simulink model "Vehicle_Model_999_Modular_roll_gradient"  (R2025b)
settings: Solver=ode23tb  StartTime=0.0  StopTime=72  MaxStep=0.001  RelTol=1e-3
values from neighbouring files (symbols this model uses):
  aero_par = struct()    [Load_aero_parameters.m]
  Ki_array = zeros(size(Vx_array))    [Torque_vectoring_workspace_lookuptable_v2.m]
  Kp_array = zeros(size(Vx_array))    [Torque_vectoring_workspace_lookuptable_v2.m]
  ku = (lr*m*9.81/(cf*(lf+lr))) - (lf*m*9.81/(cr*(lf+lr)))    (= -0.00172747958109)    [Torque_vectoring_workspace_lookuptable_v2.m]
  m = Par.m    [Lapsim_Endurance_inverse_v3.m]    (also in New_LapSim_final_ts_v1.m = Par.Mass; Rajdeep_sus_scriptv2.m = 270; Torque_vectoring_workspace_lookuptable_v2.m = 270)
  Par = struct()    [Load_vehicle_parameters.m]
  path_Theta = theta-theta_0    [New_LapSim_final_ts_v1.m]
  sus_par = struct()    [Load_sus_parameters.m]
  TireData = Tir    [prep_tire_data.m]
  Vx_array = 1:1:21    [Torque_vectoring_workspace_lookuptable_v2.m]
undefined symbols (not defined in the file or in its folder): additional_steering, Battery, Brake_Val, ctrl_Brake, ctrl_s, ctrl_Steer, ctrl_Throttle, ctrl_Velocity, HP, init_r, init_vx, init_vy, Motor, path_X, path_Y, skidpad_time, skidpad_vel, steer_input, Steer_Val, TC_target_slip, Throttle_Val, V_ref
libraries: simulink x16, autolibshared x3, simulink_extras x2, BatteryEstimators x1
(part 2 of 4)

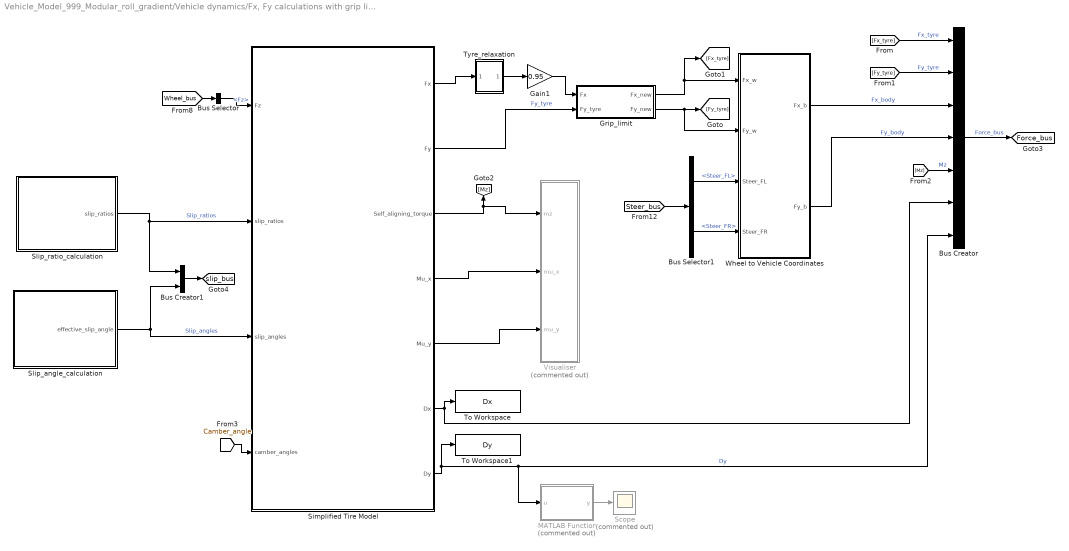
== system Vehicle_Model_999_Modular_roll_gradient/Vehicle dynamics/Fx, Fy calculations with grip limit ==
  Bus Creator : BusCreator  Inputs=7
  Bus Creator1 : BusCreator  Inputs=2
  Bus Selector : BusSelector  OutputSignals=Fz
  Bus Selector1 : BusSelector  OutputSignals=Steer_FL,Steer_FR
  Gain1 : Gain  Gain=0.95
  Grip_limit : Subsystem
  MATLAB Function : MATLAB Function  Commented=on  TreatAsAtomicUnit=on
  Scope : Scope  Commented=on
      settings: ActiveDisplayYMinimum=-1  ActiveDisplayYMaximum=1  DataLoggingVariableName=ScopeData16
  Simplified Tire Model : MATLAB Function  TreatAsAtomicUnit=on
  Slip_angle_calculation : Subsystem
  Slip_ratio_calculation : Subsystem
  To Workspace : ToWorkspace  VariableName=Dx  SaveFormat=Timeseries  SampleTime=-1
  To Workspace1 : ToWorkspace  VariableName=Dy  SaveFormat=Timeseries  SampleTime=-1
  Tyre_relaxation : Subsystem
  Visualiser : Subsystem  Commented=on
  Wheel to Vehicle Coordinates : MATLAB Function  TreatAsAtomicUnit=on
  tag scope: Force_bus=global, slip_bus=global
  wires:
  Simplified Tire Model/1(Fx) -> Tyre_relaxation/1(Fx_ss)
  Simplified Tire Model/6(Dx) -> To Workspace/1, Bus Creator/6
  [Wheel_bus] -> Bus Selector/1
  Bus Selector/1 -> Simplified Tire Model/1(Fz)  "<Fz>"
  Bus Creator1/1 -> [slip_bus]
  Bus Creator/1 -> [Force_bus]  "Force_bus"
  [Mz] -> Bus Creator/5  "Mz"
  [Fx_tyre] -> Bus Creator/1  "Fx_tyre"
  [Fy_tyre] -> Bus Creator/2  "Fy_tyre"
  Slip_ratio_calculation/1(slip_ratios) -> Simplified Tire Model/2(slip_ratios), Bus Creator1/1  "Slip_ratios"
  Slip_angle_calculation/1(effective_slip_angle) -> Simplified Tire Model/3(slip_angles), Bus Creator1/2  "Slip_angles"
  Bus Selector1/2 -> Wheel to Vehicle Coordinates/4(Steer_FR)  "<Steer_FR>"
  [Steer_bus] -> Bus Selector1/1
  Simplified Tire Model/4(Mu_x) -> Visualiser/2(mu_x)
  Wheel to Vehicle Coordinates/1(Fx_b) -> Bus Creator/3  "Fx_body"
  Simplified Tire Model/5(Mu_y) -> Visualiser/3(mu_y)
  Bus Selector1/1 -> Wheel to Vehicle Coordinates/3(Steer_FL)  "<Steer_FL>"
  Simplified Tire Model/7(Dy) -> MATLAB Function/1(u), Bus Creator/7, To Workspace1/1  "Dy"
  Tyre_relaxation/1(Fx_w) -> Gain1/1
  Simplified Tire Model/3(Self_aligning_torque) -> Visualiser/1(mz), [Mz]
  Wheel to Vehicle Coordinates/2(Fy_b) -> Bus Creator/4  "Fy_body"
  [Camber_angle] -> Simplified Tire Model/4(camber_angles)
  MATLAB Function/1(y) -> Scope/1
  Grip_limit/2(Fy_new) -> Wheel to Vehicle Coordinates/2(Fy_w), [Fy_tyre]
  Grip_limit/1(Fx_new) -> [Fx_tyre], Wheel to Vehicle Coordinates/1(Fx_w)
  Gain1/1 -> Grip_limit/1(Fx)
  Simplified Tire Model/2(Fy) -> Grip_limit/2(Fy_tyre)  "Fy_tyre"

== system Vehicle_Model_999_Modular_roll_gradient/Vehicle dynamics/Rolling and Drag forces ==
  Aero Drag : MATLAB Function  TreatAsAtomicUnit=on
  Bus Creator : BusCreator  Inputs=3
  Bus Selector : BusSelector  OutputSignals=Fz
  Bus Selector1 : BusSelector  OutputSignals=Steer_FL,Steer_FR
  Bus Selector2 : BusSelector  OutputSignals=Longitudinal_vel,Lateral_vel
  MATLAB Function : MATLAB Function  TreatAsAtomicUnit=on
  Rolling Forces : MATLAB Function  TreatAsAtomicUnit=on
  Terminator : Terminator
  To Workspace : ToWorkspace  Commented=on  VariableName=Dragforce  SaveFormat=Timeseries  SampleTime=-1
  tag scope: Resistive_force_bus=global
  wires:
  Bus Selector1/1 -> Rolling Forces/2(Steer_FL)  "<Steer_FL>"
  Bus Selector2/1 -> Aero Drag/1(vx)  "<Longitudinal_vel>"
  Bus Selector/1 -> Rolling Forces/1(Fz)  "<Fz>"
  Aero Drag/1(B_F_aero) -> MATLAB Function/1(u), Bus Creator/3  "Aero_drag_force"
  Rolling Forces/1(Fx_rr_b) -> Bus Creator/1  "Longitudinal_rolling_resistance"
  Bus Selector1/2 -> Rolling Forces/3(Steer_FR)  "<Steer_FR>"
  Bus Selector2/2 -> Aero Drag/2(vy)  "<Lateral_vel>"
  Rolling Forces/2(Fy_rr_b) -> Bus Creator/2  "Lateral_rolling_resistance"
  Bus Creator/1 -> [Resistive_force_bus]
  MATLAB Function/1(y) -> To Workspace/1, Terminator/1  "Drag_force"
  [Wheel_bus] -> Bus Selector/1
  [Steer_bus] -> Bus Selector1/1
  [chassisbus] -> Bus Selector2/1

== system Vehicle_Model_999_Modular_roll_gradient/Vehicle dynamics/Steering ==
  Bus Selector12 : BusSelector  OutputSignals=Steer_input
  Constant1 : Constant  Value=sus_par.Acc_pct
  Steering Kinematics : Subsystem
  tag scope: Steer_bus=global
  wires:
  Bus Selector12/1 -> Steering Kinematics/1(Steer_Input)  "<Steer_input>"
  Constant1/1 -> Steering Kinematics/2(Ackermann_Pct)
  [Input_bus] -> Bus Selector12/1
  Steering Kinematics/1(Steering Angles) -> [Steer_bus]

== system Vehicle_Model_999_Modular_roll_gradient/Vehicle dynamics/Steering_new ==
  Bus Creator1 : BusCreator  Inputs=2
  Bus Selector12 : BusSelector  OutputSignals=Steer_input
  Display : Display  Commented=on
  Display1 : Display  Commented=on
  Steering Kinematics : MATLAB Function  TreatAsAtomicUnit=on
  To Workspace : ToWorkspace  VariableName=steer_L  SaveFormat=Timeseries  SampleTime=-1
  To Workspace1 : ToWorkspace  VariableName=steer_R  SaveFormat=Timeseries  SampleTime=-1
  tag scope: Steer_bus=global
  wires:
  Bus Creator1/1 -> [Steer_bus]
  [Input_bus] -> Bus Selector12/1
  Bus Selector12/1 -> Steering Kinematics/1(steering_wheel_angle)  "<Steer_input>"
  Steering Kinematics/2(Steer_R) -> Display/1, To Workspace1/1, Bus Creator1/2  "Steer_FR"
  Steering Kinematics/1(Steer_L) -> Display1/1, To Workspace/1, Bus Creator1/1  "Steer_FL"

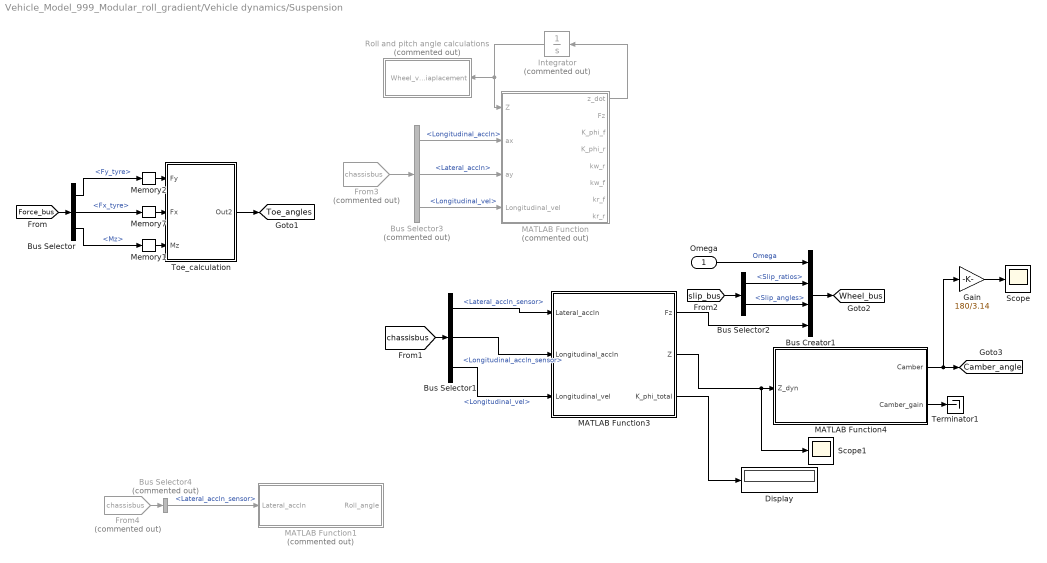
== system Vehicle_Model_999_Modular_roll_gradient/Vehicle dynamics/Suspension ==
  Omega : Inport
  Bus Creator1 : BusCreator  Inputs=4
  Bus Selector : BusSelector  OutputSignals=Fy_tyre,Fx_tyre,Mz
  Bus Selector1 : BusSelector  OutputSignals=Lateral_accln_sensor,Longitudinal_accln_sensor,Longitudinal_vel
  Bus Selector2 : BusSelector  OutputSignals=Slip_ratios,Slip_angles
  Bus Selector3 : BusSelector  Commented=on  OutputSignals=Longitudinal_accln,Lateral_accln,Longitudinal_vel
  Bus Selector4 : BusSelector  Commented=on  OutputSignals=Lateral_accln_sensor
  Display : Display
  From3 : From  Commented=on  GotoTag=chassisbus  TagVisibility=global
  From4 : From  Commented=on  GotoTag=chassisbus  TagVisibility=global
  Gain : Gain  Gain=180/3.14
  Integrator : Integrator  Commented=on
  MATLAB Function : MATLAB Function  Commented=on  TreatAsAtomicUnit=on
  MATLAB Function1 : MATLAB Function  Commented=on  TreatAsAtomicUnit=on
  MATLAB Function3 : MATLAB Function  TreatAsAtomicUnit=on
  MATLAB Function4 : MATLAB Function  TreatAsAtomicUnit=on
  Memory1 : Memory
  Memory2 : Memory
  Memory7 : Memory
  Roll and pitch angle calculations : Subsystem  Commented=on
  Scope : Scope
      settings: ActiveDisplayYMinimum=-0.32429469761940044  ActiveDisplayYMaximum=0.29371949735728869  DataLoggingVariableName=ScopeData3
  Scope1 : Scope
      settings: ActiveDisplayYMinimum=-0.021192676708042583  ActiveDisplayYMaximum=0.035474266047541975  DataLoggingVariableName=ScopeData4
  Terminator1 : Terminator
  Toe_calculation : Subsystem
  tag scope: Camber_angle=global, Toe_angles=global, Wheel_bus=global
  wires:
  Toe_calculation/1(Out2) -> [Toe_angles]
  Memory7/1 -> Toe_calculation/2(Fx)
  Memory1/1 -> Toe_calculation/3(Mz)
  Memory2/1 -> Toe_calculation/1(Fy)
  Bus Selector/1 -> Memory2/1  "<Fy_tyre>"
  [Force_bus] -> Bus Selector/1
  Bus Selector/2 -> Memory7/1  "<Fx_tyre>"
  Bus Selector/3 -> Memory1/1  "<Mz>"
  Omega/1 -> Bus Creator1/1  "Omega"
  Bus Selector2/2 -> Bus Creator1/3  "<Slip_angles>"
  From3/1 -> Bus Selector3/1
  Bus Selector3/1 -> MATLAB Function/2(ax)  "<Longitudinal_accln>"
  Bus Selector2/1 -> Bus Creator1/2  "<Slip_ratios>"
  Bus Selector3/2 -> MATLAB Function/3(ay)  "<Lateral_accln>"
  Bus Creator1/1 -> [Wheel_bus]
  [slip_bus] -> Bus Selector2/1
  Integrator/1 -> Roll and pitch angle calculations/1(Wheel_vertical_diaplacement), MATLAB Function/1(Z)
  Bus Selector3/3 -> MATLAB Function/4(Longitudinal_vel)  "<Longitudinal_vel>"
  MATLAB Function3/1(Fz) -> Bus Creator1/4
  [chassisbus] -> Bus Selector1/1
  Bus Selector1/3 -> MATLAB Function3/3(Longitudinal_vel)  "<Longitudinal_vel>"
  MATLAB Function4/1(Camber) -> Gain/1, [Camber_angle]
  MATLAB Function4/2(Camber_gain) -> Terminator1/1
  MATLAB Function3/2(Z) -> Scope1/1, MATLAB Function4/1(Z_dyn)
  MATLAB Function/1(z_dot) -> Integrator/1
  Bus Selector1/1 -> MATLAB Function3/1(Lateral_accln)  "<Lateral_accln_sensor>"
  Bus Selector1/2 -> MATLAB Function3/2(Longitudinal_accln)  "<Longitudinal_accln_sensor>"
  From4/1 -> Bus Selector4/1
  Bus Selector4/1 -> MATLAB Function1/1(Lateral_accln)  "<Lateral_accln_sensor>"
  Gain/1 -> Scope/1
  MATLAB Function3/3(K_phi_total) -> Display/1

== system Vehicle_Model_999_Modular_roll_gradient/Vehicle dynamics/Wheel_dynamics ==
  Bus Selector13 : BusSelector  OutputSignals=Fz
  Bus Selector14 : BusSelector  OutputSignals=Slip_angles
  Bus Selector30 : BusSelector  OutputSignals=Omega
  Rolling Resistance : MATLAB Function  TreatAsAtomicUnit=on
  Wheel Dynamics : Subsystem
  Omega1 : Outport
  wires:
  [Wheel_bus] -> Bus Selector14/1, Bus Selector30/1, Bus Selector13/1
  Bus Selector30/1 -> Rolling Resistance/2(Omega)  "<Omega>"
  Rolling Resistance/1(wFx_rr) -> Wheel Dynamics/1(Fx_rr)
  Bus Selector13/1 -> Rolling Resistance/1(Fz)  "<Fz>"
  Bus Selector14/1 -> Rolling Resistance/3(slip_angles)  "<Slip_angles>"
  Wheel Dynamics/1(Omega) -> Omega1/1

== system Vehicle_Model_999_Modular_roll_gradient/Visualization/Visualize Fx ==
  Fx_tire : Inport
  Demux : Demux
  To Workspace : ToWorkspace  VariableName=Longitudinal_force_fl  SaveFormat=Timeseries  SampleTime=-1
  To Workspace1 : ToWorkspace  VariableName=Longitudinal_force_fr  SaveFormat=Timeseries  SampleTime=-1
  To Workspace2 : ToWorkspace  VariableName=Longitudinal_force_rl  SaveFormat=Timeseries  SampleTime=-1
  To Workspace3 : ToWorkspace  VariableName=Longitudinal_force_rr  SaveFormat=Timeseries  SampleTime=-1
  Visualize_longitudinal_force_tire : Scope  Commented=on  NumInputPorts=4
      settings: ActiveDisplayYMinimum=-744.61831418304712  ActiveDisplayYMaximum=150.84371621033421  DataLoggingVariableName=ScopeData2
  wires:
  Fx_tire/1 -> Demux/1
  Demux/1 -> To Workspace/1, Visualize_longitudinal_force_tire/1  "Longitudinal_force_fl"
  Demux/2 -> To Workspace1/1, Visualize_longitudinal_force_tire/2  "Longitudinal_force_fr"
  Demux/3 -> To Workspace2/1, Visualize_longitudinal_force_tire/3  "Longitudinal_force_rl"
  Demux/4 -> To Workspace3/1, Visualize_longitudinal_force_tire/4  "Longitudinal_force_rr"

== system Vehicle_Model_999_Modular_roll_gradient/Visualization/Visualize Fy ==
  Fy_tire : Inport
  Demux : Demux
  To Workspace1 : ToWorkspace  VariableName=Lateral_force_fl  SaveFormat=Timeseries  SampleTime=-1
  To Workspace2 : ToWorkspace  VariableName=Lateral_force_fr  SaveFormat=Timeseries  SampleTime=-1
  To Workspace3 : ToWorkspace  VariableName=Lateral_force_rl  SaveFormat=Timeseries  SampleTime=-1
  To Workspace4 : ToWorkspace  VariableName=Lateral_force_rr  SaveFormat=Timeseries  SampleTime=-1
  Visualize_lateral_force_tire : Scope  Commented=on  NumInputPorts=4
      settings: ActiveDisplayYMinimum=-149.71186810034453  ActiveDisplayYMaximum=870.76288445594662  DataLoggingVariableName=ScopeData2
  wires:
  Demux/4 -> To Workspace4/1, Visualize_lateral_force_tire/4  "Lateral_force_rr"
  Demux/3 -> To Workspace3/1, Visualize_lateral_force_tire/3  "Lateral_force_rl"
  Demux/2 -> To Workspace2/1, Visualize_lateral_force_tire/2  "Lateral_force_fr"
  Demux/1 -> To Workspace1/1, Visualize_lateral_force_tire/1  "Lateral_force_fl"
  Fy_tire/1 -> Demux/1

== system Vehicle_Model_999_Modular_roll_gradient/Visualization/Visualize Fz ==
  Fz : Inport
  Demux : Demux
  To Workspace : ToWorkspace  VariableName=Fz  SaveFormat=Timeseries  SampleTime=-1
  Visualize_Fz : Scope  Commented=on  NumInputPorts=4
      settings: ActiveDisplayYMinimum=-105.77095780933836  ActiveDisplayYMaximum=951.93862028404544  DataLoggingVariableName=ScopeData2
  wires:
  Fz/1 -> Demux/1
  Demux/1 -> To Workspace/1, Visualize_Fz/1  "Fz_fl"
  Demux/2 -> Visualize_Fz/2  "Fz_fr"
  Demux/3 -> Visualize_Fz/3  "Fz_rl"
  Demux/4 -> Visualize_Fz/4  "Fz_rr"

== system Vehicle_Model_999_Modular_roll_gradient/E-powertrain/Battery Pack/Subsystem ==
  In1 : Inport
  Constant : Constant  Value=0.001
  Switch : Switch  Criteria=u2 > Threshold  SaturateOnIntegerOverflow=off  InputSameDT=off
  Out1 : Outport
  wires:
  In1/1 -> Switch/1, Switch/2
  Constant/1 -> Switch/3
  Switch/1 -> Out1/1

== system Vehicle_Model_999_Modular_roll_gradient/E-powertrain/Torque Distribution/Torque Vectoring ==
  steering angle : Inport
  vx : Inport  Port=2
  real yaw rate : Inport  Port=3
  Wheel Torques : Inport  Port=4
  1-D Lookup Table1 : Lookup_n-D  NumberOfTableDimensions=1  BreakpointsForDimension1=Vx_array  Table=Kp_array  InternalRulePriority=Speed  RndMeth=Simplest
  1-D Lookup Table2 : Lookup_n-D  NumberOfTableDimensions=1  BreakpointsForDimension1=Vx_array  Table=Ki_array  InternalRulePriority=Speed  RndMeth=Simplest
  MATLAB Function : MATLAB Function  TreatAsAtomicUnit=on
  MATLAB Function1 : MATLAB Function  TreatAsAtomicUnit=on
  PID controller in time domain : MATLAB Function  TreatAsAtomicUnit=on  SystemSampleTime=0.001
  Target yaw rate : Subsystem
  To Workspace : ToWorkspace  VariableName=Target_yaw_rate  SaveFormat=Timeseries  SampleTime=-1
  Vectored Torque Commands : Outport
  wires:
  steering angle/1 -> Target yaw rate/1(steering angle)
  Wheel Torques/1 -> MATLAB Function/1(wheel_torques)
  MATLAB Function/1(vectored_torques) -> Vectored Torque Commands/1
  vx/1 -> 1-D Lookup Table2/1, 1-D Lookup Table1/1, Target yaw rate/2(vx)
  PID controller in time domain/1(yaw_moment) -> MATLAB Function/2(yaw_moment)
  real yaw rate/1 -> MATLAB Function1/1(u)
  MATLAB Function1/1(y) -> PID controller in time domain/2(y)
  1-D Lookup Table1/1 -> PID controller in time domain/3(Kp)
  1-D Lookup Table2/1 -> PID controller in time domain/4(Ki)
  Target yaw rate/1(target yaw rate) -> To Workspace/1, PID controller in time domain/1(ref)

== system Vehicle_Model_999_Modular_roll_gradient/E-powertrain/Torque Distribution/Traction Control ==
  Wheel Torque : Inport
  Slip Ratios : Inport  Port=2
  vx : Inport  Port=3
  Constant3 : Constant  Value=TC_target_slip
  KD1 : Lookup_n-D  NumberOfTableDimensions=1  BreakpointsForDimension1=[0, 55e-10, 0.0045, 2, 8.5,9]  Table=[0, 0, 0.0014, 0.0109,0,0]  InternalRulePriority=Speed  RndMeth=Simplest
  KI1 : Lookup_n-D  NumberOfTableDimensions=1  BreakpointsForDimension1=[0; 55e-10;0.0045; 2; 8.5]  Table=[0.1; 0.1;700; 500; 450 ]  InternalRulePriority=Speed  RndMeth=Simplest
  KP1 : Lookup_n-D  NumberOfTableDimensions=1  BreakpointsForDimension1=[0; 55e-10; 0.0045; 2; 8.5]  Table=[ 0.5; 0.5; 2.5; 10; 10]  InternalRulePriority=Speed  RndMeth=Simplest
  MATLAB Function1 : MATLAB Function  TreatAsAtomicUnit=on  SystemSampleTime=0.001
  MATLAB Function2 : MATLAB Function  TreatAsAtomicUnit=on
  Traction Controlled Torque : Outport
  wires:
  KD1/1 -> MATLAB Function1/5(Kd)
  KI1/1 -> MATLAB Function1/4(Ki)
  KP1/1 -> MATLAB Function1/3(Kp)
  vx/1 -> KD1/1, KI1/1, KP1/1
  Slip Ratios/1 -> MATLAB Function1/2(lambda_actual)
  Constant3/1 -> MATLAB Function1/1(lambda_ref)
  Wheel Torque/1 -> MATLAB Function2/2(torque_wheel)
  MATLAB Function1/1(throttle_cmd) -> MATLAB Function2/1(torque_pid)
  MATLAB Function2/1(TC_output) -> Traction Controlled Torque/1

== system Vehicle_Model_999_Modular_roll_gradient/E-powertrain/Torque Distribution/is TCS on? ==
  traction_controlled_torque : Inport
  In1 : Inport  Port=2
  TV_T_wheel : Inport  Port=3
  AND : Logic  IconShape=distinctive  AllPortsSameDT=off  OutDataTypeStr=boolean
  Bus Selector6 : BusSelector  OutputSignals=Steer_input
  MATLAB Function1 : MATLAB Function  TreatAsAtomicUnit=on
  Switch : Switch  Criteria=u2 > Threshold  SaturateOnIntegerOverflow=off  InputSameDT=off
  torque_output : Outport
  wires:
  Switch/1 -> torque_output/1
  TV_T_wheel/1 -> Switch/3
  traction_controlled_torque/1 -> Switch/1
  In1/1 -> AND/2
  AND/1 -> Switch/2
  Bus Selector6/1 -> MATLAB Function1/1(Steer_input)  "<Steer_input>"
  [Input_bus] -> Bus Selector6/1
  MATLAB Function1/1(TC_on) -> AND/1

== system Vehicle_Model_999_Modular_roll_gradient/E-powertrain/Torque Distribution/is TV on? ==
  vectored_torque : Inport
  In1 : Inport  Port=2
  wheel_torque : Inport  Port=3
  Switch : Switch  Criteria=u2 > Threshold  SaturateOnIntegerOverflow=off  InputSameDT=off
  torque_output : Outport
  wires:
  wheel_torque/1 -> Switch/3
  vectored_torque/1 -> Switch/1
  Switch/1 -> torque_output/1
  In1/1 -> Switch/2

== system Vehicle_Model_999_Modular_roll_gradient/Inputs/Brake_input_selector/Brake Variant Subsystem ==
  brake_sim : Inport
  vel : Inport  Port=2
  GGV : Subsystem  VariantControl=Mode_ggv
  Sideslip_vs_curvature_cst_accln : Subsystem  VariantControl=Mode_sideslip_vs_curvature_cst_accln
  Simulink : Subsystem  VariantControl=Mode_simulink
  curvature vs steer_angle : Subsystem  VariantControl=Mode_curvature_vs_steer
  sideslip_vs_curvature : Subsystem  VariantControl=Mode_sideslip_vs_curvature
  steerdiff_vs_ay : Subsystem  VariantControl=Mode_steerdiff_vs_ay
  timeseries : Subsystem  VariantControl=Mode_timeseries
  brake_input : Outport
  accln : Outport  Port=2

== system Vehicle_Model_999_Modular_roll_gradient/Inputs/Subsystem/Subsystem ==
  In1 : Inport
  Abs : Abs  SaturateOnIntegerOverflow=off
  Constant : Constant  Value=0.0001
  Switch : Switch  Criteria=u2 > Threshold  SaturateOnIntegerOverflow=off  InputSameDT=off
  Out1 : Outport
  wires:
  In1/1 -> Abs/1, Switch/1
  Constant/1 -> Switch/3
  Abs/1 -> Switch/2
  Switch/1 -> Out1/1

== system Vehicle_Model_999_Modular_roll_gradient/Inputs/Subsystem/Subsystem1 ==
  In1 : Inport
  Abs : Abs  SaturateOnIntegerOverflow=off
  Constant : Constant  Value=0.0001
  Switch : Switch  Criteria=u2 > Threshold  SaturateOnIntegerOverflow=off  InputSameDT=off
  Out1 : Outport
  wires:
  In1/1 -> Abs/1, Switch/1
  Constant/1 -> Switch/3
  Abs/1 -> Switch/2
  Switch/1 -> Out1/1

== system Vehicle_Model_999_Modular_roll_gradient/Inputs/Subsystem/Triggered Subsystem ==
  In1 : Inport
  Trigger : TriggerPort  VariantControl=(inherit)
  Out1 : Outport
  wires:
  In1/1 -> Out1/1

== system Vehicle_Model_999_Modular_roll_gradient/Inputs/Subsystem/Triggered Subsystem1 ==
  In1 : Inport
  Trigger : TriggerPort  VariantControl=(inherit)
  Out1 : Outport
  wires:
  In1/1 -> Out1/1

== system Vehicle_Model_999_Modular_roll_gradient/Inputs/Subsystem/Triggered Subsystem2 ==
  In1 : Inport
  Trigger : TriggerPort  VariantControl=(inherit)
  Out1 : Outport
  wires:
  In1/1 -> Out1/1

== system Vehicle_Model_999_Modular_roll_gradient/Inputs/Subsystem/Triggered Subsystem3 ==
  In1 : Inport
  In3 : Inport  Port=2
  Trigger : TriggerPort  VariantControl=(inherit)
  Out1 : Outport
  Out3 : Outport  Port=2
  wires:
  In1/1 -> Out1/1
  In3/1 -> Out3/1

== system Vehicle_Model_999_Modular_roll_gradient/Inputs/Subsystem/Triggered Subsystem4 ==
  In1 : Inport
  Trigger : TriggerPort  VariantControl=(inherit)
  Out1 : Outport
  wires:
  In1/1 -> Out1/1

== system Vehicle_Model_999_Modular_roll_gradient/Inputs/Subsystem/Triggered Subsystem5 ==
  In1 : Inport
  Trigger : TriggerPort  VariantControl=(inherit)
  Out1 : Outport
  wires:
  In1/1 -> Out1/1

== system Vehicle_Model_999_Modular_roll_gradient/Inputs/Subsystem/Triggered Subsystem6 ==
  In1 : Inport
  Trigger : TriggerPort  VariantControl=(inherit)
  Out1 : Outport
  wires:
  In1/1 -> Out1/1

== system Vehicle_Model_999_Modular_roll_gradient/Inputs/Subsystem1/Triggered Subsystem ==
  In1 : Inport
  Trigger : TriggerPort  VariantControl=(inherit)
  Out1 : Outport
  wires:
  In1/1 -> Out1/1

== system Vehicle_Model_999_Modular_roll_gradient/Inputs/Subsystem1/Triggered Subsystem1 ==
  In1 : Inport
  Trigger : TriggerPort  VariantControl=(inherit)
  Out1 : Outport
  wires:
  In1/1 -> Out1/1

== system Vehicle_Model_999_Modular_roll_gradient/Inputs/Subsystem1/Triggered Subsystem2 ==
  In1 : Inport
  Trigger : TriggerPort  VariantControl=(inherit)
  Out1 : Outport
  wires:
  In1/1 -> Out1/1

== system Vehicle_Model_999_Modular_roll_gradient/Inputs/Throttle_input_selector/Throttle Variant Subsystem ==
  accln : Inport
  accln_input_for_map1 : Inport  Port=2
  GGV : Subsystem  VariantControl=Mode_ggv
  Simulink : Subsystem  VariantControl=Mode_simulink
  Timeseries : Subsystem  VariantControl=Mode_timeseries
  curvature vs steer : Subsystem  VariantControl=Mode_curvature_vs_steer
  sideslip_vs_curvature : Subsystem  VariantControl=Mode_sideslip_vs_curvature
  sideslip_vs_curvature_cst_accln : Subsystem  VariantControl=Mode_sideslip_vs_curvature_cst_accln
  steerdiff_vs_ay : Subsystem  VariantControl=Mode_steerdiff_vs_ay
  throttle : Outport

== system Vehicle_Model_999_Modular_roll_gradient/Inputs/steer_input_selector/Steering Variant Subsystem ==
  In1 : Inport
  GGV : Subsystem  VariantControl=Mode_ggv
  Simulink : Subsystem  VariantControl=Mode_simulink
  Timeseries : Subsystem  VariantControl=Mode_timeseries
  curvature_vs_steering_angle : Subsystem  VariantControl=Mode_curvature_vs_steer
  sideslip_vs_curvature_1 : Subsystem  VariantControl=Mode_sideslip_vs_curvature
  sideslip_vs_curvature_constant_lat_accln : Subsystem  VariantControl=Mode_sideslip_vs_curvature_cst_accln
  steerdiff_vs_ay : Subsystem  VariantControl=Mode_steerdiff_vs_ay
  Steer Input : Outport

== system Vehicle_Model_999_Modular_roll_gradient/Vehicle dynamics/Force and Torque Equilibrium/Subsystem ==
  In1 : Inport
  Clock : Clock
  Compare To Constant : simulink/Logic and Bit Operations/Compare To Constant  relop=>=  const=75  OutDataTypeStr=boolean
  Detect Rise Positive : simulink/Logic and Bit Operations/Detect Rise Positive  vinit=0  OutDataTypeStr=boolean
  Triggered Subsystem : Subsystem  TreatAsAtomicUnit=on
  Out1 : Outport
  wires:
  In1/1 -> Compare To Constant/1
  Detect Rise Positive/1 -> Triggered Subsystem/Trigger
  Clock/1 -> Triggered Subsystem/1(In1)
  Triggered Subsystem/1(Out1) -> Out1/1
  Compare To Constant/1 -> Detect Rise Positive/1

== system Vehicle_Model_999_Modular_roll_gradient/Vehicle dynamics/Force and Torque Equilibrium/Subsystem1 ==
  In1 : Inport
  Constant : Constant  Value=0.001
  Switch : Switch  Criteria=u2 > Threshold  SaturateOnIntegerOverflow=off  InputSameDT=off
  Out1 : Outport
  wires:
  In1/1 -> Switch/1, Switch/2
  Constant/1 -> Switch/3
  Switch/1 -> Out1/1

== system Vehicle_Model_999_Modular_roll_gradient/Vehicle dynamics/Force and Torque Equilibrium/Visualize Fx ==
  Fx_body : Inport
  Demux : Demux
  To Workspace : ToWorkspace  VariableName=Longitudinal_force_body_fl  SaveFormat=Timeseries  SampleTime=-1
  To Workspace1 : ToWorkspace  VariableName=Longitudinal_force_body_fr  SaveFormat=Timeseries  SampleTime=-1
  To Workspace2 : ToWorkspace  VariableName=Longitudinal_force_body_rl  SaveFormat=Timeseries  SampleTime=-1
  To Workspace3 : ToWorkspace  VariableName=Longitudinal_force_body_rr  SaveFormat=Timeseries  SampleTime=-1
  Visualize_longitudinal_force_body : Scope  Commented=on  NumInputPorts=4
      settings: ActiveDisplayYMinimum=-1  ActiveDisplayYMaximum=1  DataLoggingVariableName=ScopeData2
  wires:
  Fx_body/1 -> Demux/1
  Demux/1 -> To Workspace/1, Visualize_longitudinal_force_body/1  "Longitudinal_force_fl"
  Demux/2 -> To Workspace1/1, Visualize_longitudinal_force_body/2  "Longitudinal_force_fr"
  Demux/3 -> To Workspace2/1, Visualize_longitudinal_force_body/3  "Longitudinal_force_rl"
  Demux/4 -> To Workspace3/1, Visualize_longitudinal_force_body/4  "Longitudinal_force_rr"

== system Vehicle_Model_999_Modular_roll_gradient/Vehicle dynamics/Force and Torque Equilibrium/Visualize Fy ==
  Fy_tire : Inport
  Demux : Demux
  To Workspace1 : ToWorkspace  VariableName=Lateral_force_body_fl  SaveFormat=Timeseries  SampleTime=-1
  To Workspace2 : ToWorkspace  VariableName=Lateral_force_body_fr  SaveFormat=Timeseries  SampleTime=-1
  To Workspace3 : ToWorkspace  VariableName=Lateral_force_body_rl  SaveFormat=Timeseries  SampleTime=-1
  To Workspace4 : ToWorkspace  VariableName=Lateral_force_body_rr  SaveFormat=Timeseries  SampleTime=-1
  Visualize_lateral_force_body : Scope  Commented=on  NumInputPorts=4
      settings: ActiveDisplayYMinimum=-1  ActiveDisplayYMaximum=1  DataLoggingVariableName=ScopeData2
  wires:
  Demux/4 -> To Workspace4/1, Visualize_lateral_force_body/4  "Lateral_force_rr"
  Demux/3 -> To Workspace3/1, Visualize_lateral_force_body/3  "Lateral_force_rl"
  Demux/2 -> To Workspace2/1, Visualize_lateral_force_body/2  "Lateral_force_fr"
  Demux/1 -> To Workspace1/1, Visualize_lateral_force_body/1  "Lateral_force_fl"
  Fy_tire/1 -> Demux/1

== system Vehicle_Model_999_Modular_roll_gradient/Vehicle dynamics/Fx, Fy calculations with grip limit/Grip_limit ==
  Fx : Inport
  Fy_tyre : Inport  Port=2
  Bus Selector2 : BusSelector  OutputSignals=Dx,Dy
  Bus Selector3 : BusSelector  OutputSignals=Longitudinal_disp
  MATLAB Function1 : MATLAB Function  TreatAsAtomicUnit=on
  Fx_new : Outport
  Fy_new : Outport  Port=2
  wires:
  Bus Selector2/2 -> MATLAB Function1/4(Dy)  "<Dy>"
  Bus Selector3/1 -> MATLAB Function1/5(s)  "<Longitudinal_disp>"
  Bus Selector2/1 -> MATLAB Function1/3(Dx)  "<Dx>"
  [chassisbus] -> Bus Selector3/1
  [Force_bus] -> Bus Selector2/1
  MATLAB Function1/1(Fx_new) -> Fx_new/1
  Fy_tyre/1 -> MATLAB Function1/2(Fy)
  Fx/1 -> MATLAB Function1/1(Fx)
  MATLAB Function1/2(Fy_new) -> Fy_new/1

== system Vehicle_Model_999_Modular_roll_gradient/Vehicle dynamics/Fx, Fy calculations with grip limit/Slip_angle_calculation ==
  Bus Selector25 : BusSelector  OutputSignals=Longitudinal_vel
  Bus Selector26 : BusSelector  OutputSignals=Lateral_vel
  Bus Selector27 : BusSelector  OutputSignals=Yaw_rate
  Bus Selector28 : BusSelector  OutputSignals=Steer_FL
  Bus Selector29 : BusSelector  OutputSignals=Steer_FR
  Slip Angles : MATLAB Function  TreatAsAtomicUnit=on
  Subsystem : Subsystem
  Visualize Slip_angle : Subsystem  Commented=on
  effective_slip_angle : Outport
  wires:
  [Toe_angles] -> Subsystem/1(toe)
  Subsystem/1(slip_ratio) -> effective_slip_angle/1, Visualize Slip_angle/1(slip_angle)  "effective_slip_angle"
  Bus Selector29/1 -> Slip Angles/5(Steer_FR)  "<Steer_FR>"
  Bus Selector28/1 -> Slip Angles/4(Steer_FL)  "<Steer_FL>"
  Slip Angles/1(slip_angles) -> Subsystem/2(slip_angles)
  Bus Selector25/1 -> Slip Angles/1(Longitudinal_vel)  "<Longitudinal_vel>"
  [chassisbus] -> Bus Selector25/1, Bus Selector26/1, Bus Selector27/1
  [Steer_bus] -> Bus Selector28/1, Bus Selector29/1
  Bus Selector27/1 -> Slip Angles/3(yawrate)  "<Yaw_rate>"
  Bus Selector26/1 -> Slip Angles/2(Lateral_vel)  "<Lateral_vel>"

== system Vehicle_Model_999_Modular_roll_gradient/Vehicle dynamics/Fx, Fy calculations with grip limit/Slip_ratio_calculation ==
  Bus Selector21 : BusSelector  OutputSignals=Longitudinal_vel
  Bus Selector22 : BusSelector  OutputSignals=Yaw_rate
  Bus Selector23 : BusSelector  OutputSignals=Omega
  Bus Selector24 : BusSelector  OutputSignals=Lateral_vel
  Bus Selector32 : BusSelector  OutputSignals=Steer_FL
  Bus Selector33 : BusSelector  OutputSignals=Steer_FR
  Visualize Slip_ratios : Subsystem  Commented=on
  slip ratios : MATLAB Function  TreatAsAtomicUnit=on
  slip_ratios : Outport
  wires:
  slip ratios/1(slip_ratios) -> slip_ratios/1, Visualize Slip_ratios/1(slip_ratio)  "slip_ratios"
  [Wheel_bus] -> Bus Selector23/1
  Bus Selector24/1 -> slip ratios/2(Vy)  "<Lateral_vel>"
  Bus Selector33/1 -> slip ratios/6(Steer_FR)  "<Steer_FR>"
  Bus Selector22/1 -> slip ratios/3(yawrate)  "<Yaw_rate>"
  [chassisbus] -> Bus Selector21/1, Bus Selector24/1, Bus Selector22/1
  Bus Selector32/1 -> slip ratios/5(Steer_FL)  "<Steer_FL>"
  Bus Selector23/1 -> slip ratios/4(Omega)  "<Omega>"
  Bus Selector21/1 -> slip ratios/1(Vx)  "<Longitudinal_vel>"
  [Steer_bus] -> Bus Selector33/1, Bus Selector32/1

== system Vehicle_Model_999_Modular_roll_gradient/Vehicle dynamics/Fx, Fy calculations with grip limit/Tyre_relaxation ==
  Fx_ss : Inport
  Bus Selector : BusSelector  OutputSignals=Longitudinal_vel
  Integrator : Integrator
  MATLAB Function : MATLAB Function  TreatAsAtomicUnit=on
  Fx_w : Outport
  wires:
  [chassisbus] -> Bus Selector/1
  Bus Selector/1 -> MATLAB Function/3(Vx)  "<Longitudinal_vel>"
  Integrator/1 -> MATLAB Function/2(Fx_act), Fx_w/1
  MATLAB Function/1(Fx_dot) -> Integrator/1
  Fx_ss/1 -> MATLAB Function/1(Fx_ss)

== system Vehicle_Model_999_Modular_roll_gradient/Vehicle dynamics/Fx, Fy calculations with grip limit/Visualiser ==
  mz : Inport
  mu_x : Inport  Port=2
  mu_y : Inport  Port=3
  Demux : Demux
  Demux1 : Demux
  Demux2 : Demux
  Scope : Scope  NumInputPorts=4
  Scope1 : Scope  NumInputPorts=4
  Scope2 : Scope  NumInputPorts=4
  wires:
  Demux2/4 -> Scope2/4
  Demux2/1 -> Scope2/1
  mu_y/1 -> Demux2/1
  Demux2/2 -> Scope2/2
  Demux2/3 -> Scope2/3
  Demux1/4 -> Scope1/4
  Demux1/1 -> Scope1/1
  mu_x/1 -> Demux1/1
  Demux1/2 -> Scope1/2
  Demux1/3 -> Scope1/3
  Demux/4 -> Scope/4
  Demux/3 -> Scope/3
  Demux/2 -> Scope/2
  Demux/1 -> Scope/1
  mz/1 -> Demux/1

== system Vehicle_Model_999_Modular_roll_gradient/Vehicle dynamics/Steering/Steering Kinematics ==
  Steer_Input : Inport
  Ackermann_Pct : Inport  Port=2
  Bus Creator1 : BusCreator  Inputs=2
  Display : Display
  Display1 : Display
  Gain : Gain  Gain=180/pi
  Gain1 : Gain  Gain=180/pi
  Steering Kinematics : MATLAB Function  TreatAsAtomicUnit=on
  To Workspace : ToWorkspace  VariableName=steer_L  SaveFormat=Timeseries  SampleTime=-1
  To Workspace1 : ToWorkspace  VariableName=steer_R  SaveFormat=Timeseries  SampleTime=-1
  Steering Angles : Outport
  wires:
  Steering Kinematics/1(Steer_FL) -> To Workspace/1, Gain/1, Bus Creator1/1  "Steer_FL"
  Steer_Input/1 -> Steering Kinematics/1(Steer_Input)
  Steering Kinematics/2(Steer_FR) -> To Workspace1/1, Gain1/1, Bus Creator1/2  "Steer_FR"
  Ackermann_Pct/1 -> Steering Kinematics/2(Ackermann_Pct)
  Bus Creator1/1 -> Steering Angles/1
  Gain/1 -> Display1/1
  Gain1/1 -> Display/1

== system Vehicle_Model_999_Modular_roll_gradient/Vehicle dynamics/Suspension/Roll and pitch angle calculations ==
  Wheel_vertical_diaplacement : Inport
  Gain : Gain  Gain=180/pi
  Gain1 : Gain  Gain=180/pi
  Pitch_angle_calcualtions : MATLAB Function  TreatAsAtomicUnit=on
  Roll_angle_calulations : MATLAB Function  TreatAsAtomicUnit=on
  Scope : Scope  NumInputPorts=2
      settings: ActiveDisplayYMinimum=-0.14321062822354433  ActiveDisplayYMaximum=0.97414830718088607  DataLoggingVariableName=ScopeData11
  To Workspace : ToWorkspace  VariableName=roll_angle  SaveFormat=Timeseries  SampleTime=-1
  wires:
  Wheel_vertical_diaplacement/1 -> Pitch_angle_calcualtions/1(z_wheel), Roll_angle_calulations/1(z_wheel)
  Pitch_angle_calcualtions/1(Pitch_angle) -> Gain/1
  Roll_angle_calulations/1(Roll_angle) -> Gain1/1
  Gain1/1 -> Scope/2, To Workspace/1
  Gain/1 -> Scope/1

== system Vehicle_Model_999_Modular_roll_gradient/Vehicle dynamics/Suspension/Toe_calculation ==
  Fy : Inport
  Fx : Inport  Port=2
  Mz : Inport  Port=3
  Mux1 : Mux
  toe_fl1 : MATLAB Function  TreatAsAtomicUnit=on
  Out2 : Outport
  wires:
  Mux1/1 -> Out2/1
  Mz/1 -> toe_fl1/3(Mz)
  Fx/1 -> toe_fl1/2(Fx_tire)
  Fy/1 -> toe_fl1/1(Fy_tire)
  toe_fl1/1(Toe_fl) -> Mux1/1
  toe_fl1/2(Toe_fr) -> Mux1/2
  toe_fl1/3(Toe_rl) -> Mux1/3
  toe_fl1/4(Toe_rr) -> Mux1/4

== system Vehicle_Model_999_Modular_roll_gradient/Vehicle dynamics/Wheel_dynamics/Wheel Dynamics ==
  Fx_rr : Inport
  Bus Selector8 : BusSelector  OutputSignals=Fx_tyre
  Integrator : Integrator  InitialCondition=init_vx/Par.R0  LimitOutput=on  UpperSaturationLimit=1e6
  MATLAB Function : MATLAB Function  TreatAsAtomicUnit=on
  MATLAB Function1 : MATLAB Function  Commented=on  TreatAsAtomicUnit=on
  Omega : Outport
  wires:
  [Torque_inputs] -> MATLAB Function/1(T_in)
  Fx_rr/1 -> MATLAB Function/2(Fx_rr)
  MATLAB Function/1(Omega_dot) -> Integrator/1
  [Force_bus] -> Bus Selector8/1
  Bus Selector8/1 -> MATLAB Function/3(Fx_tire)  "<Fx_tyre>"
  Integrator/1 -> Omega/1, MATLAB Function/4(Omega)

== system Vehicle_Model_999_Modular_roll_gradient/E-powertrain/Torque Distribution/Torque Vectoring/Target yaw rate ==
  steering angle : Inport
  vx : Inport  Port=2
  Bus Selector : BusSelector  OutputSignals=Dy
  Bus Selector1 : BusSelector  OutputSignals=Fz
  MATLAB Function : MATLAB Function  TreatAsAtomicUnit=on
  target yaw rate : Outport
  ideal_yaw : Outport  Port=2
  wires:
  vx/1 -> MATLAB Function/1(vx)
  steering angle/1 -> MATLAB Function/2(delta)
  MATLAB Function/1(target_yaw) -> target yaw rate/1
  MATLAB Function/2(ideal_yaw) -> ideal_yaw/1
  [Force_bus] -> Bus Selector/1
  [Wheel_bus] -> Bus Selector1/1
  Bus Selector1/1 -> MATLAB Function/3(Fz)  "<Fz>"
  Bus Selector/1 -> MATLAB Function/4(Dy)  "<Dy>"

== system Vehicle_Model_999_Modular_roll_gradient/Inputs/Brake_input_selector/Brake Variant Subsystem/GGV ==
  Constant : Constant  Value=Brake_Val
  brake_input : Outport
  wires:
  Constant/1 -> brake_input/1

== system Vehicle_Model_999_Modular_roll_gradient/Inputs/Brake_input_selector/Brake Variant Subsystem/Sideslip_vs_curvature_cst_accln ==
  vel : Inport
  Constant : Constant  Value=10
  Constant3 : Constant  Value=0
  Longitudinal Driver : autolibshared/Longitudinal Driver  extAccelOvr=off  extDecelOvr=off  extAccelHld=off  extDecelHld=off  extAccelZero=off  extDecelZero=off  cntrlType=PI  shftType=None  velUnits=m/s  gearOut=off  Kp=10  Ki=5  Kff=.1  Kg=0  VehVelVec=[0 100]  KffVec=[.1 .1]  KpVec=[10 10]  KiVec=[5 5]  KgVec=[0 0]  m=1500  Kpt=3000  tau=.1  L=2  aR=200  bR=2.5  cR=.5  g=9.81  vnom=5  Kaw=1  tauerr=.01  tauPt=2  GearInit=0  tShift=.1  pdlVec=[0.1 0.4 0.5 0.9]  upShftTbl=[-1 12.9375 26.4375 39.9375 51.18749999999999 62.4375 72.84375 83.25;-1 16.3125 29.8125 43.3125 54.5624 65.8125 76.78125 87.75;-1 19.6875 33.1875 46.68749999999999 57.9375 69.1875 80.71875 92.25;-1 33 52.5 77.25 100.5 138.75 161.875 185]  dwnShftTbl=[1 9.5625 23.0625 36.5625 47.8125 59.0625 68.90625 78.75;1 12.9375 26.4375 39.9375 51.18749999999999 62.4375 72.84375 83.25;1 16.3125 29.8125 43.3125 54.562499 65.8125 76.78125 87.75;1 19.6875 33.1875 46.68749999999999 57.9375 69.1875 80.71875 92.25]  tClutch=.5  tRev=.5  tPark=120  aMode=2  UpGearVec="[0  1  2  3  4  5  6  7]"  DownGearVec="[1  2  3  4  5  6  7  8]"
      settings: LibrarySourceBlock=vehdynlibdriver/Longitudinal Driver
  Terminator1 : Terminator
  brake_input : Outport
  accln : Outport  Port=2
  wires:
  Constant3/1 -> Longitudinal Driver/3
  Constant/1 -> Longitudinal Driver/1
  Longitudinal Driver/1 -> Terminator1/1
  Longitudinal Driver/2 -> accln/1
  Longitudinal Driver/3 -> brake_input/1
  vel/1 -> Longitudinal Driver/2

== system Vehicle_Model_999_Modular_roll_gradient/Inputs/Brake_input_selector/Brake Variant Subsystem/Simulink ==
  brake_sim : Inport
  brake_input : Outport
  wires:
  brake_sim/1 -> brake_input/1

== system Vehicle_Model_999_Modular_roll_gradient/Inputs/Brake_input_selector/Brake Variant Subsystem/curvature vs steer_angle ==
  vel : Inport
  Constant : Constant  Value=V_ref
  Constant3 : Constant  Value=0
  Longitudinal Driver : autolibshared/Longitudinal Driver  extAccelOvr=off  extDecelOvr=off  extAccelHld=off  extDecelHld=off  extAccelZero=off  extDecelZero=off  cntrlType=PI  shftType=None  velUnits=m/s  gearOut=off  Kp=10  Ki=5  Kff=.1  Kg=0  VehVelVec=[0 100]  KffVec=[.1 .1]  KpVec=[10 10]  KiVec=[5 5]  KgVec=[0 0]  m=1500  Kpt=3000  tau=.1  L=2  aR=200  bR=2.5  cR=.5  g=9.81  vnom=5  Kaw=1  tauerr=.01  tauPt=2  GearInit=0  tShift=.1  pdlVec=[0.1 0.4 0.5 0.9]  upShftTbl=[-1 12.9375 26.4375 39.9375 51.18749999999999 62.4375 72.84375 83.25;-1 16.3125 29.8125 43.3125 54.5624 65.8125 76.78125 87.75;-1 19.6875 33.1875 46.68749999999999 57.9375 69.1875 80.71875 92.25;-1 33 52.5 77.25 100.5 138.75 161.875 185]  dwnShftTbl=[1 9.5625 23.0625 36.5625 47.8125 59.0625 68.90625 78.75;1 12.9375 26.4375 39.9375 51.18749999999999 62.4375 72.84375 83.25;1 16.3125 29.8125 43.3125 54.562499 65.8125 76.78125 87.75;1 19.6875 33.1875 46.68749999999999 57.9375 69.1875 80.71875 92.25]  tClutch=.5  tRev=.5  tPark=120  aMode=2  UpGearVec="[0  1  2  3  4  5  6  7]"  DownGearVec="[1  2  3  4  5  6  7  8]"
      settings: LibrarySourceBlock=vehdynlibdriver/Longitudinal Driver
  Terminator : Terminator
  brake_input : Outport
  accln : Outport  Port=2
  wires:
  Longitudinal Driver/3 -> brake_input/1
  Constant3/1 -> Longitudinal Driver/3
  Longitudinal Driver/1 -> Terminator/1
  Constant/1 -> Longitudinal Driver/1
  Longitudinal Driver/2 -> accln/1
  vel/1 -> Longitudinal Driver/2

== system Vehicle_Model_999_Modular_roll_gradient/Inputs/Brake_input_selector/Brake Variant Subsystem/sideslip_vs_curvature ==
  brake_sim : Inport
  brake_input : Outport
  wires:
  brake_sim/1 -> brake_input/1

== system Vehicle_Model_999_Modular_roll_gradient/Inputs/Brake_input_selector/Brake Variant Subsystem/steerdiff_vs_ay ==
  Constant : Constant  Value=0
  brake_input : Outport
  wires:
  Constant/1 -> brake_input/1

== system Vehicle_Model_999_Modular_roll_gradient/Inputs/Brake_input_selector/Brake Variant Subsystem/timeseries ==
  From Workspace : FromWorkspace  VariableName=brake_ts
  brake_input : Outport
  wires:
  From Workspace/1 -> brake_input/1

== system Vehicle_Model_999_Modular_roll_gradient/Inputs/Throttle_input_selector/Throttle Variant Subsystem/GGV ==
  SimInput_Throttle : Constant  Value=Throttle_Val
  throttle : Outport
  wires:
  SimInput_Throttle/1 -> throttle/1

== system Vehicle_Model_999_Modular_roll_gradient/Inputs/Throttle_input_selector/Throttle Variant Subsystem/Simulink ==
  accln : Inport
  throttle : Outport
  wires:
  accln/1 -> throttle/1

== system Vehicle_Model_999_Modular_roll_gradient/Inputs/Throttle_input_selector/Throttle Variant Subsystem/Timeseries ==
  From Workspace : FromWorkspace  VariableName=throttle_ts
  throttle : Outport
  wires:
  From Workspace/1 -> throttle/1

== system Vehicle_Model_999_Modular_roll_gradient/Inputs/Throttle_input_selector/Throttle Variant Subsystem/curvature vs steer ==
  accln_input_for_map1 : Inport
  throttle : Outport
  wires:
  accln_input_for_map1/1 -> throttle/1

== system Vehicle_Model_999_Modular_roll_gradient/Inputs/Throttle_input_selector/Throttle Variant Subsystem/sideslip_vs_curvature ==
  Constant : Constant
  throttle : Outport
  wires:
  Constant/1 -> throttle/1

== system Vehicle_Model_999_Modular_roll_gradient/Inputs/Throttle_input_selector/Throttle Variant Subsystem/sideslip_vs_curvature_cst_accln ==
  accln_input_for_map1 : Inport
  throttle : Outport
  wires:
  accln_input_for_map1/1 -> throttle/1

== system Vehicle_Model_999_Modular_roll_gradient/Inputs/Throttle_input_selector/Throttle Variant Subsystem/steerdiff_vs_ay ==
  Clock : Clock
  Constant1 : Constant  Value=0.25
  Ramp : simulink/Sources/Ramp  slope=2  start=0  InitialOutput=0
  Saturation : Saturate  UpperLimit=1  LowerLimit=0
  Switch : Switch  Criteria=u2 > Threshold  Threshold=4  SaturateOnIntegerOverflow=off  InputSameDT=off
  throttle : Outport
  wires:
  Clock/1 -> Switch/2
  Ramp/1 -> Switch/3
  Switch/1 -> Saturation/1
  Constant1/1 -> Switch/1
  Saturation/1 -> throttle/1

== system Vehicle_Model_999_Modular_roll_gradient/Inputs/steer_input_selector/Steering Variant Subsystem/GGV ==
  SimInput_Steer : Constant  Value=Steer_Val
  Steer Input : Outport
  wires:
  SimInput_Steer/1 -> Steer Input/1

== system Vehicle_Model_999_Modular_roll_gradient/Inputs/steer_input_selector/Steering Variant Subsystem/Simulink ==
  In1 : Inport
  Steer Input : Outport
  wires:
  In1/1 -> Steer Input/1

== system Vehicle_Model_999_Modular_roll_gradient/Inputs/steer_input_selector/Steering Variant Subsystem/Timeseries ==
  From Workspace : FromWorkspace  VariableName=steer_ts
  Steer Input : Outport
  wires:
  From Workspace/1 -> Steer Input/1

== system Vehicle_Model_999_Modular_roll_gradient/Inputs/steer_input_selector/Steering Variant Subsystem/curvature_vs_steering_angle ==
  Clock1 : Clock
  Constant1 : Constant  Value=0
  Ramp2 : simulink/Sources/Ramp  slope=pi/60  start=10  InitialOutput=0
  Saturation1 : Saturate  UpperLimit=pi/6
  Switch1 : Switch  Criteria=u2 > Threshold  Threshold=10  SaturateOnIntegerOverflow=off  InputSameDT=off
  Steer Input : Outport
  wires:
  Switch1/1 -> Saturation1/1
  Ramp2/1 -> Switch1/1
  Clock1/1 -> Switch1/2
  Constant1/1 -> Switch1/3
  Saturation1/1 -> Steer Input/1

== system Vehicle_Model_999_Modular_roll_gradient/Inputs/steer_input_selector/Steering Variant Subsystem/sideslip_vs_curvature_1 ==
  Clock : Clock
  Constant : Constant  Value=0
  Constant1 : Constant  Value=steer_input
  Saturation : Saturate  UpperLimit=pi/20
  Switch : Switch  Criteria=u2 > Threshold  Threshold=4  SaturateOnIntegerOverflow=off  InputSameDT=off
  Steer Input : Outport
  wires:
  Switch/1 -> Saturation/1
  Saturation/1 -> Steer Input/1
  Constant1/1 -> Switch/1
  Clock/1 -> Switch/2
  Constant/1 -> Switch/3

== system Vehicle_Model_999_Modular_roll_gradient/Inputs/steer_input_selector/Steering Variant Subsystem/sideslip_vs_curvature_constant_lat_accln ==
  Clock : Clock
  Constant : Constant  Value=0
  Ramp : simulink/Sources/Ramp  slope=pi/100  start=4  InitialOutput=0
  Saturation : Saturate  UpperLimit=pi/20
  Switch : Switch  Criteria=u2 > Threshold  Threshold=4  SaturateOnIntegerOverflow=off  InputSameDT=off
  Steer Input : Outport
  wires:
  Switch/1 -> Saturation/1
  Saturation/1 -> Steer Input/1
  Ramp/1 -> Switch/1
  Clock/1 -> Switch/2
  Constant/1 -> Switch/3

== system Vehicle_Model_999_Modular_roll_gradient/Inputs/steer_input_selector/Steering Variant Subsystem/steerdiff_vs_ay ==
  Clock : Clock
  Constant : Constant  Value=0
  Ramp : simulink/Sources/Ramp  slope=pi/30  start=5  InitialOutput=0
  Saturation : Saturate  UpperLimit=pi/6  LowerLimit=0
  Switch : Switch  Criteria=u2 > Threshold  Threshold=5  SaturateOnIntegerOverflow=off  InputSameDT=off
  Steer Input : Outport
  wires:
  Switch/1 -> Saturation/1
  Ramp/1 -> Switch/1
  Constant/1 -> Switch/3
  Clock/1 -> Switch/2
  Saturation/1 -> Steer Input/1

== system Vehicle_Model_999_Modular_roll_gradient/Vehicle dynamics/Force and Torque Equilibrium/Subsystem/Triggered Subsystem ==
  In1 : Inport
  Trigger : TriggerPort  VariantControl=(inherit)
  Out1 : Outport
  wires:
  In1/1 -> Out1/1

== system Vehicle_Model_999_Modular_roll_gradient/Vehicle dynamics/Fx, Fy calculations with grip limit/Slip_angle_calculation/Subsystem ==
  toe : Inport
  slip_angles : Inport  Port=2
  Subtract : Sum  Inputs=+-
  slip_ratio : Outport
  wires:
  Subtract/1 -> slip_ratio/1
  toe/1 -> Subtract/2
  slip_angles/1 -> Subtract/1

== system Vehicle_Model_999_Modular_roll_gradient/Vehicle dynamics/Fx, Fy calculations with grip limit/Slip_angle_calculation/Visualize Slip_angle ==
  slip_angle : Inport
  Demux : Demux
  To Workspace : ToWorkspace  VariableName=slip_angle_fl  SaveFormat=Timeseries  SampleTime=-1
  To Workspace1 : ToWorkspace  VariableName=slip_angle_fr  SaveFormat=Timeseries  SampleTime=-1
  To Workspace2 : ToWorkspace  VariableName=slip_angle_rl  SaveFormat=Timeseries  SampleTime=-1
  To Workspace3 : ToWorkspace  VariableName=slip_angle_rr  SaveFormat=Timeseries  SampleTime=-1
  Visualize_slip_angle : Scope  NumInputPorts=4
      settings: ActiveDisplayYMinimum=-1  ActiveDisplayYMaximum=1  DataLoggingVariableName=ScopeData2
  wires:
  Demux/4 -> Visualize_slip_angle/4, To Workspace3/1  "slip_angle_rr"
  Demux/3 -> Visualize_slip_angle/3, To Workspace2/1  "slip_angle_rl"
  Demux/2 -> Visualize_slip_angle/2, To Workspace1/1  "slip_angle_fr"
  Demux/1 -> Visualize_slip_angle/1, To Workspace/1  "slip_angle_fl"
  slip_angle/1 -> Demux/1

== system Vehicle_Model_999_Modular_roll_gradient/Vehicle dynamics/Fx, Fy calculations with grip limit/Slip_ratio_calculation/Visualize Slip_ratios ==
  slip_ratio : Inport
  Demux : Demux
  To Workspace : ToWorkspace  VariableName=slip_ratio_fl  SaveFormat=Timeseries  SampleTime=-1
  To Workspace1 : ToWorkspace  VariableName=slip_ratio_fr  SaveFormat=Timeseries  SampleTime=-1
  To Workspace2 : ToWorkspace  VariableName=slip_ratio_rl  SaveFormat=Timeseries  SampleTime=-1
  To Workspace3 : ToWorkspace  VariableName=slip_ratio_rr  SaveFormat=Timeseries  SampleTime=-1
  Visualize_slip_ratio : Scope  NumInputPorts=4
      settings: ActiveDisplayYMinimum=-1  ActiveDisplayYMaximum=1  DataLoggingVariableName=ScopeData2
  wires:
  Demux/4 -> To Workspace3/1, Visualize_slip_ratio/4  "slip_ratio_rr"
  Demux/3 -> To Workspace2/1, Visualize_slip_ratio/3  "slip_ratio_rl"
  Demux/2 -> To Workspace1/1, Visualize_slip_ratio/2  "slip_ratio_fr"
  Demux/1 -> Visualize_slip_ratio/1, To Workspace/1  "slip_ratio_fl"
  slip_ratio/1 -> Demux/1

== matlab function Vehicle_Model_999_Modular_roll_gradient/Vehicle dynamics/Wheel_dynamics/Wheel Dynamics/MATLAB Function ==
  data: T_in input; Omega_dot output; Fx_rr input; Fx_tire input; Omega input; Par parameter; Motor parameter
function Omega_dot = fcn(T_in, Fx_rr, Fx_tire, Omega, Par,Motor)
%#codegen
    
    % 1. Enforce Column Vectors (Protects against array dimension mismatch)
    T_in = T_in(:);
    Fx_rr = Fx_rr(:);
    Fx_tire = Fx_tire(:);
    Omega = Omega(:);
    
    % 2. Constants
    R = Par.R0;
    Iw = Par.Iw;
    
    % Assuming your parameters struct now contains the max speed limit
    % Define this in your workspace script: Par.Omega_max = Motor.n_max * 2 * pi / (60 * 10.05);
    Omega_max = Motor.n_max * 2 * pi / (60 * 10.05); 
    
    % Rotational damping parameter
    b_w = 0.1; 
    
    % 3. Separate Drive and Brake capacities
    % Note: Assumes T_in > 0 is forward drive, T_in < 0 is braking. 
    T_drive = max(T_in, 0); 
    T_brake_capacity = abs(min(T_in, 0)); 
    
    % Smooth directional multiplier to avoid zero-crossing step discontinuities
    Rotation_Dir = tanh(10 .* Omega);
    
    % 4. Calculate external torques BEFORE brakes are applied
    T_tire_reaction = abs(Fx_rr .* R) .* Rotation_Dir;
    T_tire = Fx_tire .* R;
    T_damping = b_w .* Omega;
    
    % Net torque tending to move the wheel
    T_pre_brake = T_drive - T_tire_reaction - T_tire - T_damping;
    
    % 5. Continuous Blended Brake Logic
    T_brake_dynamic = -T_brake_capacity .* Rotation_Dir;
    T_brake_static = -max(min(T_pre_brake, T_brake_capacity), -T_brake_capacity);
    
    % Blend factor: approaches 0 when stopped, approaches 1 when moving
    moving_flag = abs(tanh(10 .* Omega));
    
    % Final applied brake torque
    T_brake_actual = (moving_flag .* T_brake_dynamic) + ((1 - moving_flag) .* T_brake_static);
    
    % 6. Compute Raw Angular Acceleration
    T_net = T_pre_brake + T_brake_actual;
    Omega_dot_raw = T_net ./ Iw;
    
    % =====================================================================
    % 7. STATE DERIVATIVE LIMITING (Anti-Windup)
    % =====================================================================
    % Start with the raw acceleration
    Omega_dot = Omega_dot_raw;
    
    % Condition 1: Wheel is at or above max speed AND torque is trying to accelerate it further.
    % We clamp the derivative to 0 to prevent it from exceeding the limit.
    at_pos_limit = (Omega >= Omega_max) & (Omega_dot_raw > 0);
    Omega_dot(at_pos_limit) = 0;
    
    % Condition 2 (Optional but recommended): Reverse speed limit.
    % Prevents the wheel from over-speeding in reverse.
    at_neg_limit = (Omega <= -Omega_max) & (Omega_dot_raw < 0);
    Omega_dot(at_neg_limit) = 0;

end

== matlab function Vehicle_Model_999_Modular_roll_gradient/Inputs/MATLAB Function ==
  data: ideal_ref_vel input; y output; skidpad_vel input
function y = fcn(ideal_ref_vel,skidpad_vel)

y = max(ideal_ref_vel,5);
% y = 1.193*max(ideal_ref_vel,1.5);
% R = 9.125;
% y = 2*pi*R/skidpad_time;
% y = skidpad_vel;
% y = 12.5;
